simulink library "CCM_FVT"  (R2024a)
settings: Solver=VariableStepAuto  StartTime=0.0  StopTime=10.0  RelTol=1e-3
undefined symbols (not defined in the file or in its folder): ACCM_facCCMLq_X_A, ACCM_facCCMLq_Y_A, ACCM_facLPFiDAct_X_rpm, ACCM_IdKp_X_rpm, ACCM_tiCurErrOvr_X_A, CCM_bRstIpartTrig_C, CCM_bRstPIMor_C, CCM_bRstPITrig_C, CCM_bUseCCMVolFFTrig_C, CCM_bUseUvw_flg, CCM_facAngleComp, CCM_facCCMKiUdTar_T, CCM_facCCMKiUqTar_T, CCM_facCCMKpUdTar_T, CCM_facCCMKpUqTar_T, CCM_facCCMLd_T, CCM_facCCMLq_T, CCM_facLPFiDAct_T, CCM_facLPFiQAct_T, CCM_iCurrDQRstIntgl_C, CCM_iDCurrAct_A, CCM_iDErrDeadZoneLo_C, CCM_iDErrDeadZoneUp_C, CCM_iQErrDeadZoneLo_C, CCM_iQErrDeadZoneUp_C, CCM_nRotCCMKpKi_A, CCM_nRotRstIntgl_C, CCM_nRotSpdLPFiDQAct_A, CCM_uDVoltTarMax_C, CCM_uDVoltTarMin_C, CCM_uDVoltTarMor_C, CCM_uDVoltTarTrig_C, CCM_uQVoltTarMax_C, CCM_uQVoltTarMin_C, CCM_uQVoltTarMor_C, CCM_uQVoltTarTrig_C, CDC_iQCurrAct_A, CDC_tqMotCurrTarMTPV_A, ENUM_IVTROPMODE_DTCYCTRL, IvtrM_vVehPCM2SpdKpKiTar_A, KCCM_BattVolFilTi_fac, KCCM_bRstCurErrorOverThd_C, KCCM_CurLoopPrd_t, KCCM_FwdMask_c, KCCM_IdKi_null, KCCM_IdKp_null, KCCM_IdKt_null, KCCM_IqKi_null, KCCM_IqKp_null, KCCM_IqKt_null, KCCM_PosnRange_deg, KCCM_tiCurErrOvr_C, KCCM_UdqASCEna_C, KCCM_UdqASCTagValue_C, KCCM_UdqASCTimesValue_C, KCCM_VdSp_V, KCCM_VdSpSwEna_flg, KCCM_VolMod_perc, KCCM_VqSp_V, KDSM_CurErrorThd2_value ... (+33)
libraries: simulink x10, GRC_Lib x6, FVTMCU_lib x2
(part 1 of 2)
settings Model: Creator=FVT22063  LastModifiedBy=FVT22063

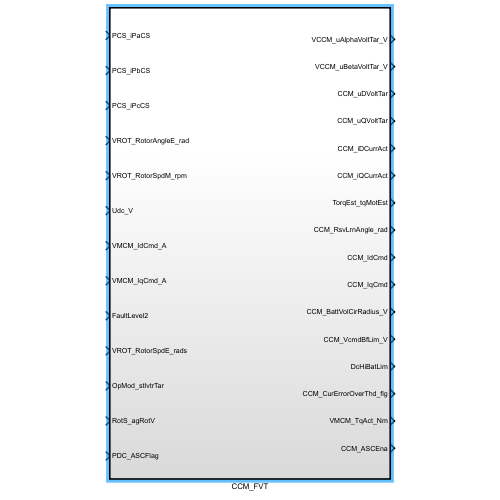
[thumbnail: Simulink's stored preview of the top-level diagram]
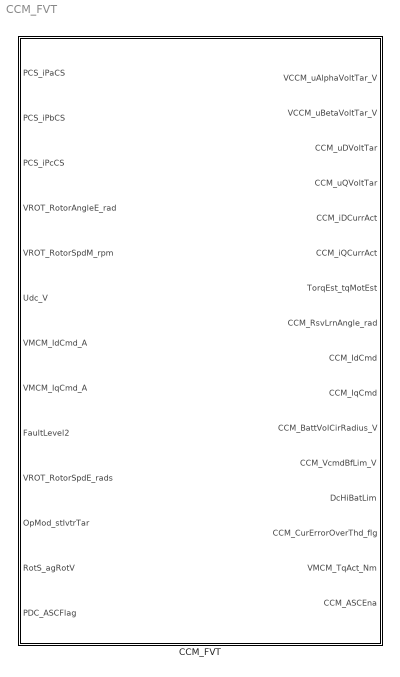
== system CCM_FVT ==
  CCM_FVT : Subsystem  TreatAsAtomicUnit=on
      settings: RTWSystemCode=Nonreusable function  RTWFcnNameOpts=Use subsystem name  RTWFileNameOpts=Use subsystem name

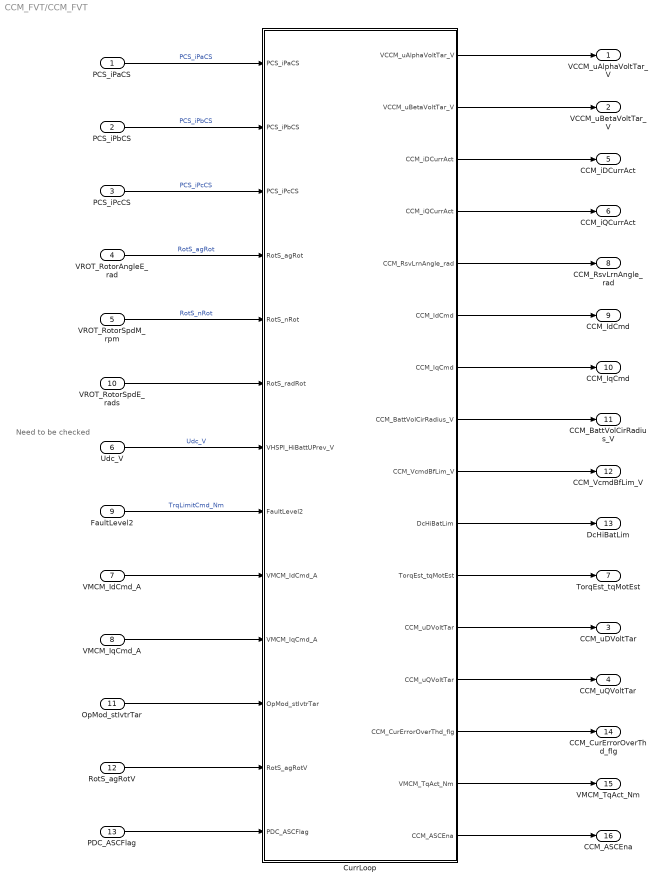
== system CCM_FVT/CCM_FVT ==
  note: Need to be checked
  PCS_iPaCS : Inport
  PCS_iPbCS : Inport  Port=2
  PCS_iPcCS : Inport  Port=3
  VROT_RotorAngleE_rad : Inport  Port=4
  VROT_RotorSpdM_rpm : Inport  Port=5
  Udc_V : Inport  Port=6
  VMCM_IdCmd_A : Inport  Port=7
  VMCM_IqCmd_A : Inport  Port=8
  FaultLevel2 : Inport  Port=9
  VROT_RotorSpdE_rads : Inport  Port=10
  OpMod_stIvtrTar : Inport  Port=11
  RotS_agRotV : Inport  Port=12
  PDC_ASCFlag : Inport  Port=13
  CurrLoop : Subsystem
  VCCM_uAlphaVoltTar_V : Outport  VectorParamsAs1DForOutWhenUnconnected=off
  VCCM_uBetaVoltTar_V : Outport  Port=2  VectorParamsAs1DForOutWhenUnconnected=off
  CCM_uDVoltTar : Outport  Port=3  VectorParamsAs1DForOutWhenUnconnected=off
  CCM_uQVoltTar : Outport  Port=4  VectorParamsAs1DForOutWhenUnconnected=off
  CCM_iDCurrAct : Outport  Port=5  VectorParamsAs1DForOutWhenUnconnected=off
  CCM_iQCurrAct : Outport  Port=6  VectorParamsAs1DForOutWhenUnconnected=off
  TorqEst_tqMotEst : Outport  Port=7  VectorParamsAs1DForOutWhenUnconnected=off
  CCM_RsvLrnAngle_rad : Outport  Port=8
  CCM_IdCmd : Outport  Port=9  VectorParamsAs1DForOutWhenUnconnected=off
  CCM_IqCmd : Outport  Port=10  VectorParamsAs1DForOutWhenUnconnected=off
  CCM_BattVolCirRadius_V : Outport  Port=11  VectorParamsAs1DForOutWhenUnconnected=off
  CCM_VcmdBfLim_V : Outport  Port=12  VectorParamsAs1DForOutWhenUnconnected=off
  DcHiBatLim : Outport  Port=13  VectorParamsAs1DForOutWhenUnconnected=off
  CCM_CurErrorOverThd_flg : Outport  Port=14  VectorParamsAs1DForOutWhenUnconnected=off
  VMCM_TqAct_Nm : Outport  Port=15  VectorParamsAs1DForOutWhenUnconnected=off
  CCM_ASCEna : Outport  Port=16  VectorParamsAs1DForOutWhenUnconnected=off
  wires:
  PCS_iPaCS/1 -> CurrLoop/1(PCS_iPaCS)  "PCS_iPaCS"
  PCS_iPbCS/1 -> CurrLoop/2(PCS_iPbCS)  "PCS_iPbCS"
  PCS_iPcCS/1 -> CurrLoop/3(PCS_iPcCS)  "PCS_iPcCS"
  VROT_RotorAngleE_rad/1 -> CurrLoop/4(RotS_agRot)  "RotS_agRot"
  VROT_RotorSpdM_rpm/1 -> CurrLoop/5(RotS_nRot)  "RotS_nRot"
  VROT_RotorSpdE_rads/1 -> CurrLoop/6(RotS_radRot)
  Udc_V/1 -> CurrLoop/7(VHSPI_HiBattUPrev_V)  "Udc_V"
  CurrLoop/1(VCCM_uAlphaVoltTar_V) -> VCCM_uAlphaVoltTar_V/1
  CurrLoop/2(VCCM_uBetaVoltTar_V) -> VCCM_uBetaVoltTar_V/1
  CurrLoop/3(CCM_iDCurrAct) -> CCM_iDCurrAct/1
  CurrLoop/4(CCM_iQCurrAct) -> CCM_iQCurrAct/1
  CurrLoop/5(CCM_RsvLrnAngle_rad) -> CCM_RsvLrnAngle_rad/1
  CurrLoop/6(CCM_IdCmd) -> CCM_IdCmd/1
  CurrLoop/7(CCM_IqCmd) -> CCM_IqCmd/1
  CurrLoop/11(TorqEst_tqMotEst) -> TorqEst_tqMotEst/1
  CurrLoop/12(CCM_uDVoltTar) -> CCM_uDVoltTar/1
  CurrLoop/13(CCM_uQVoltTar) -> CCM_uQVoltTar/1
  FaultLevel2/1 -> CurrLoop/8(FaultLevel2)  "TrqLimitCmd_Nm"
  VMCM_IdCmd_A/1 -> CurrLoop/9(VMCM_IdCmd_A)
  VMCM_IqCmd_A/1 -> CurrLoop/10(VMCM_IqCmd_A)
  OpMod_stIvtrTar/1 -> CurrLoop/11("OpMod_stIvtrTar ")
  RotS_agRotV/1 -> CurrLoop/12(RotS_agRotV)
  PDC_ASCFlag/1 -> CurrLoop/13("PDC_ASCFlag ")
  CurrLoop/8(CCM_BattVolCirRadius_V) -> CCM_BattVolCirRadius_V/1
  CurrLoop/9(CCM_VcmdBfLim_V) -> CCM_VcmdBfLim_V/1
  CurrLoop/10(DcHiBatLim) -> DcHiBatLim/1
  CurrLoop/14(CCM_CurErrorOverThd_flg) -> CCM_CurErrorOverThd_flg/1
  CurrLoop/15(VMCM_TqAct_Nm) -> VMCM_TqAct_Nm/1
  CurrLoop/16("CCM_ASCEna ") -> CCM_ASCEna/1

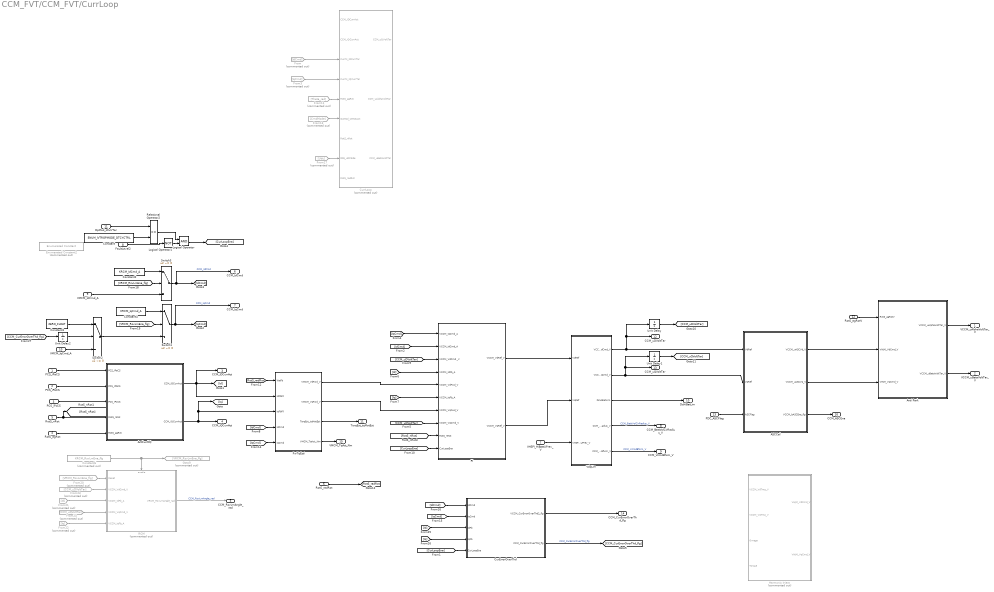
== system CCM_FVT/CCM_FVT/CurrLoop ==
  PCS_iPaCS : Inport  OutDataTypeStr=single
  PCS_iPbCS : Inport  Port=2  OutDataTypeStr=single
  PCS_iPcCS : Inport  Port=3  OutDataTypeStr=single
  RotS_agRot : Inport  Port=4  OutDataTypeStr=single
  RotS_nRot : Inport  Port=5  OutDataTypeStr=single
  RotS_radRot : Inport  Port=6
  VHSPI_HiBattUPrev_V : Inport  Port=7  OutDataTypeStr=single
  FaultLevel2 : Inport  Port=8
  VMCM_IdCmd_A : Inport  Port=9  OutDataTypeStr=single
  VMCM_IqCmd_A : Inport  Port=10  OutDataTypeStr=single
  "OpMod_stIvtrTar " : Inport  Port=11
  RotS_agRotV : Inport  Port=12  OutDataTypeStr=single
  "PDC_ASCFlag " : Inport  Port=13
  ASCCal : Subsystem
  ActCurrDQ : Subsystem
  Anti Park : Subsystem
  Constant : Constant  Value=ENUM_IVTROPMODE_DTCYCTRL
  Constant2 : Constant  Value=KRCM_IdCmd_A
  Constant3 : Constant  Value=ZERO_FLOAT
  Constant4 : Constant  Value=KRCM_IqCmd_A
  Constant6 : Constant  Commented=on  Value=KRCM_RsvLrnEna_flg  SampleTime=-1
  CurErrorOverThd : Subsystem
  CurrLoop : Subsystem  Commented=on
  Enumerated Constant2 : simulink/Sources/Enumerated Constant  Commented=on  OutDataTypeStr=Enum: StIvtrMod  Value=StIvtrMod.StIvtrModDtcyCtrl  SampleTime=inf
  From : From  Commented=on  GotoTag=IdCmd
  From11 : From  Commented=on  GotoTag=Theta_rad
  From13 : From  Commented=on  GotoTag=CmdMode
  From17 : From  Commented=on  GotoTag=Udc
  From20 : From  Commented=on  GotoTag=VRCM_RsvLrnEna_flg
  From21 : From  Commented=on  GotoTag=Id
  From22 : From  Commented=on  GotoTag=Iq
  From23 : From  Commented=on  GotoTag=CCM_uDVoltTar
  From24 : From  Commented=on  GotoTag=CCM_uQVoltTar
  From3 : From  Commented=on  GotoTag=IqCmd
  FwTqEsti : Subsystem
  Goto9 : Goto  Commented=on  GotoTag=VRCM_RsvLrnEna_flg
  Harmonic Inject : Subsystem  Commented=on
  Logical Operator : Logic  AllPortsSameDT=off  OutDataTypeStr=boolean
  Logical Operator1 : Logic  Operator=NOT  AllPortsSameDT=off  OutDataTypeStr=boolean
  PI : Subsystem
  RCM : Subsystem  Commented=on
  Relational Operator2 : RelationalOperator  Operator===  OutDataTypeStr=boolean  RndMeth=Simplest  InputSameDT=off
  Switch1 : Switch  Criteria=u2 ~= 0  SaturateOnIntegerOverflow=off  InputSameDT=off
  Switch2 : Switch  Criteria=u2 ~= 0  SaturateOnIntegerOverflow=off  InputSameDT=off
  Switch3 : Switch  Criteria=u2 ~= 0  SaturateOnIntegerOverflow=off  InputSameDT=off
  Unit Delay : UnitDelay  SampleTime=-1  HasFrameUpgradeWarning=on
  Unit Delay1 : UnitDelay  SampleTime=-1  HasFrameUpgradeWarning=on
  Unit Delay2 : UnitDelay  SampleTime=-1  HasFrameUpgradeWarning=on
  VdqLim : Subsystem
  VCCM_uAlphaVoltTar_V : Outport  OutDataTypeStr=single  VectorParamsAs1DForOutWhenUnconnected=off
  VCCM_uBetaVoltTar_V : Outport  Port=2  OutDataTypeStr=single  VectorParamsAs1DForOutWhenUnconnected=off
  CCM_iDCurrAct : Outport  Port=3  OutDataTypeStr=single  VectorParamsAs1DForOutWhenUnconnected=off
  CCM_iQCurrAct : Outport  Port=4  OutDataTypeStr=single  VectorParamsAs1DForOutWhenUnconnected=off
  CCM_RsvLrnAngle_rad : Outport  Port=5  OutDataTypeStr=single
  CCM_IdCmd : Outport  Port=6  OutDataTypeStr=single  VectorParamsAs1DForOutWhenUnconnected=off
  CCM_IqCmd : Outport  Port=7  OutDataTypeStr=single  VectorParamsAs1DForOutWhenUnconnected=off
  CCM_BattVolCirRadius_V : Outport  Port=8  OutDataTypeStr=single
  CCM_VcmdBfLim_V : Outport  Port=9  OutDataTypeStr=single
  DcHiBatLim : Outport  Port=10
  TorqEst_tqMotEst : Outport  Port=11  OutDataTypeStr=single  VectorParamsAs1DForOutWhenUnconnected=off
  CCM_uDVoltTar : Outport  Port=12  VectorParamsAs1DForOutWhenUnconnected=off
  CCM_uQVoltTar : Outport  Port=13  VectorParamsAs1DForOutWhenUnconnected=off
  CCM_CurErrorOverThd_flg : Outport  Port=14  VectorParamsAs1DForOutWhenUnconnected=off
  VMCM_TqAct_Nm : Outport  Port=15
  "CCM_ASCEna " : Outport  Port=16  VectorParamsAs1DForOutWhenUnconnected=off
  wires:
  PCS_iPaCS/1 -> ActCurrDQ/1(PCS_iPaCS)
  PCS_iPbCS/1 -> ActCurrDQ/2(PCS_iPbCS)
  PCS_iPcCS/1 -> ActCurrDQ/3(PCS_iPcCS)
  RotS_agRot/1 -> ActCurrDQ/5(RotS_agRot)
  RotS_nRot/1 -> [RotS_nRot], ActCurrDQ/4(RotS_nRot)
  From13/1 -> CurrLoop/6(OpMod_stMotAct)
  From/1 -> CurrLoop/3(CurrM_iDCurrTar)
  From3/1 -> CurrLoop/4(CurrM_iQCurrTar)
  [RotS_nRot] -> PI/9(RotS_nRot)
  From11/1 -> CurrLoop/5(RotS_agRot)
  Switch1/1 -> CCM_IqCmd/1, [IqCmd]  "CCM_IqCmd"
  From17/1 -> CurrLoop/8(DSS_uDCSide)
  Switch3/1 -> CCM_IdCmd/1, [IdCmd]  "CCM_IdCmd"
  Constant2/1 -> Switch3/1
  [VRCM_RsvLrnEna_flg] -> Switch3/2
  [VRCM_RsvLrnEna_flg] -> Switch1/2
  Constant4/1 -> Switch1/1
  Constant6/1 -> Goto9/1, RCM/Enable
  From20/1 -> RCM/1("Reset ")
  From22/1 -> RCM/5("VCCM_IqFb_A ")
  From21/1 -> RCM/3("VCCM_IdFb_A ")
  From23/1 -> RCM/2("VCCM_VdCmd_V ")
  From24/1 -> RCM/4("VCCM_VqCmd_V ")
  Unit Delay/1 -> [CCM_uDVoltTar]
  Unit Delay1/1 -> [CCM_uQVoltTar]
  RCM/1("VRCM_RsvLrnAngle_rad ") -> CCM_RsvLrnAngle_rad/1  "CCM_RsvLrnAngle_rad"
  PI/1(VCCM_VdRef_V) -> VdqLim/1(VdRef)
  VdqLim/4(CCM_BattVolCirRadius_V) -> CCM_BattVolCirRadius_V/1  "CCM_BattVolCirRadius_V"
  PI/2(VCCM_VqRef_V) -> VdqLim/2(VqRef)
  VdqLim/5(CCM_VcmdBfLim_V) -> CCM_VcmdBfLim_V/1  "CCM_VcmdBfLim_V"
  VdqLim/2(VCCM_VqCmd_V) -> ASCCal/2(VqRef), Unit Delay1/1, CCM_uQVoltTar/1
  VHSPI_HiBattUPrev_V/1 -> VdqLim/3(VHSPI_HiBattUPrev_V)
  ActCurrDQ/1(CCM_iDCurrAct) -> FwTqEsti/2(IdFbFil), [Id], CCM_iDCurrAct/1
  ActCurrDQ/2(CCM_iQCurrAct) -> [Iq], FwTqEsti/3(IqFbFil), CCM_iQCurrAct/1
  [IdCmd] -> PI/2(VCCM_IdCmd_A)
  [IqCmd] -> PI/1(VCCM_IqCmd_A)
  VMCM_IdCmd_A/1 -> Switch3/3
  RotS_radRot/1 -> [RotS_radRot]
  "OpMod_stIvtrTar "/1 -> Relational Operator2/1
  VdqLim/3(DcHiBatLim) -> DcHiBatLim/1
  RotS_agRotV/1 -> Anti Park/1(RotS_agRotV)
  Anti Park/1(VCCM_uAlphaVoltTar_V) -> VCCM_uAlphaVoltTar_V/1
  Anti Park/2(VCCM_uBetaVoltTar_V) -> VCCM_uBetaVoltTar_V/1
  VdqLim/1(VCCM_VdCmd_V) -> Unit Delay/1, CCM_uDVoltTar/1, ASCCal/1(VdRef)
  [Id] -> PI/4(VCCM_IdFb_A)
  [Iq] -> PI/6(VCCM_IqFb_A)
  [CCM_uDVoltTar] -> PI/3(VCCM_VdCmd _V)
  [CCM_uQVoltTar] -> PI/8(VCCM_VqCmd_V)
  FaultLevel2/1 -> Logical Operator1/1
  [RotS_radRot] -> FwTqEsti/1(WeFb)
  FwTqEsti/1(VMCM_VdFwd_V) -> PI/5(VCCM_VdFwd_V)
  FwTqEsti/2(VMCM_VqFwd_V) -> PI/7(VCCM_VqFwd_V)
  [IdCmd] -> FwTqEsti/4(IdCmd)
  [IqCmd] -> FwTqEsti/5(IqCmd)
  FwTqEsti/3(TorqEst_tqMotEst) -> TorqEst_tqMotEst/1
  Relational Operator2/1 -> Logical Operator/1
  Logical Operator1/1 -> Logical Operator/2
  Logical Operator/1 -> [CurLoopEna]
  [CurLoopEna] -> CurErrorOverThd/5(CurLoopEna)
  [CurLoopEna] -> PI/10(CurLoopEna)
  [IdCmd] -> CurErrorOverThd/1(IdCmd)
  [IqCmd] -> CurErrorOverThd/2(IqCmd)
  [Iq] -> CurErrorOverThd/4(IqFb)
  [Id] -> CurErrorOverThd/3(IdFb)
  FwTqEsti/4(VMCM_TqAct_Nm) -> VMCM_TqAct_Nm/1
  ASCCal/1(VCCM_uASCVd_V) -> Anti Park/2(VHJM_VdCmd_V)
  ASCCal/2(VCCM_uASCVq_V) -> Anti Park/3(VHJM_VqCmd_V)
  ASCCal/3("VCCM_bASCEna_flg ") -> "CCM_ASCEna "/1
  "PDC_ASCFlag "/1 -> ASCCal/3("ASCFlag ")
  Constant/1 -> Relational Operator2/2
  Unit Delay2/1 -> Switch2/2
  [CCM_CurErrorOverThd_flg] -> Unit Delay2/1
  Constant3/1 -> Switch2/1
  VMCM_IqCmd_A/1 -> Switch2/3
  Switch2/1 -> Switch1/3
  CurErrorOverThd/1(VCCM_CurErrorOverThd2_flg) -> CCM_CurErrorOverThd_flg/1
  CurErrorOverThd/2(CCM_CurErrorOverThd_flg) -> [CCM_CurErrorOverThd_flg]  "CCM_CurErrorOverThd_flg"

== system CCM_FVT/CCM_FVT/CurrLoop/ASCCal ==
  VdRef : Inport
  VqRef : Inport  Port=2
  "ASCFlag " : Inport  Port=3
  Constant2 : Constant  Value=KCCM_UdqASCEna_C
  If : If  IfExpression=u1 ~= 0
  If Action Subsystem : Subsystem  TreatAsAtomicUnit=on
  Merge : Merge
  Merge1 : Merge
  Merge2 : Merge
  Signal Conversion : SignalConversion  OverrideOpt=off
  Subsystem1 : Subsystem
  VCCM_uASCVd_V : Outport
  VCCM_uASCVq_V : Outport  Port=2
  "VCCM_bASCEna_flg " : Outport  Port=3
  wires:
  VqRef/1 -> If Action Subsystem/2(VqRef), Subsystem1/2(VqRef)
  Constant2/1 -> If/1
  VdRef/1 -> If Action Subsystem/1(VdRef), Subsystem1/1(VdRef)
  Merge/1 -> VCCM_uASCVd_V/1  "VCCM_uASCVd_V"
  Merge2/1 -> Signal Conversion/1  "CCM_bASCEna"
  Merge1/1 -> VCCM_uASCVq_V/1  "VCCM_uASCVq_V"
  "ASCFlag "/1 -> If Action Subsystem/3(ASCFlag), Subsystem1/3("ASCFlag ")
  If/1 -> Subsystem1/Action
  If/2 -> If Action Subsystem/Action
  If Action Subsystem/3(enASC_flg) -> Merge2/2
  If Action Subsystem/2(Vq) -> Merge1/2
  If Action Subsystem/1(Vd) -> Merge/2
  Subsystem1/3(enASC_flg) -> Merge2/1
  Subsystem1/2(Vq) -> Merge1/1
  Subsystem1/1(Vd) -> Merge/1
  Signal Conversion/1 -> "VCCM_bASCEna_flg "/1  "VCCM_bASCEna_flg"

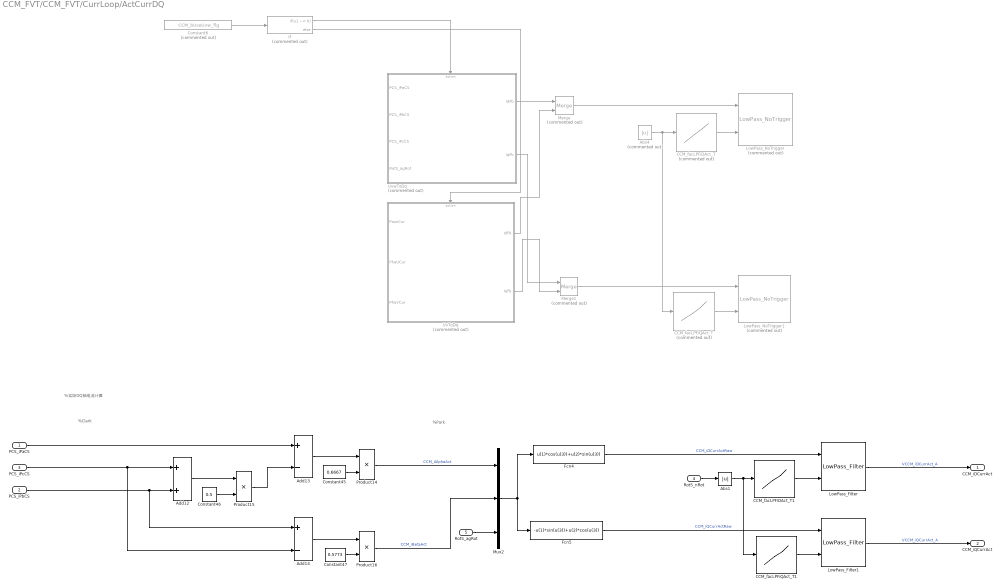
== system CCM_FVT/CCM_FVT/CurrLoop/ActCurrDQ ==
  note: %Clark
  note: %Park
  note: %实际DQ轴电流计算
  PCS_iPaCS : Inport  OutDataTypeStr=single
  PCS_iPbCS : Inport  Port=2  OutDataTypeStr=single
  PCS_iPcCS : Inport  Port=3  OutDataTypeStr=single
  RotS_nRot : Inport  Port=4  OutDataTypeStr=single
  RotS_agRot : Inport  Port=5  OutDataTypeStr=single
  Abs1 : Abs  SaturateOnIntegerOverflow=off
  Abs4 : Abs  Commented=on  SaturateOnIntegerOverflow=off
  Add12 : Sum
  Add13 : Sum  Inputs=+-
  Add14 : Sum  Inputs=+-
  CCM_facLPFiDAct_T : Lookup_n-D  Commented=on  NumberOfTableDimensions=1  BreakpointsForDimension1=CCM_nRotSpdLPFiDQAct_A  BreakpointsForDimension2=IvtrM_vVehPCM2SpdKpKiTar_A  Table=CCM_facLPFiDAct_T  TableDataTypeStr=Inherit: Inherit from 'Table data'  ExtrapMethod=Clip  UseLastTableValue=on  InternalRulePriority=Speed  OutDataTypeStr=Inherit: Inherit from 'Table data'  RndMeth=Simplest  InputSameDT=off
  CCM_facLPFiDAct_T1 : Lookup_n-D  NumberOfTableDimensions=1  BreakpointsForDimension1=ACCM_facLPFiDAct_X_rpm  BreakpointsForDimension2=IvtrM_vVehPCM2SpdKpKiTar_A  Table=MCCM_facLPFiDAct_Y_T  TableDataTypeStr=Inherit: Inherit from 'Table data'  ExtrapMethod=Clip  UseLastTableValue=on  InternalRulePriority=Speed  OutDataTypeStr=Inherit: Inherit from 'Table data'  RndMeth=Simplest  InputSameDT=off
  CCM_facLPFiQAct_T : Lookup_n-D  Commented=on  NumberOfTableDimensions=1  BreakpointsForDimension1=CCM_nRotSpdLPFiDQAct_A  BreakpointsForDimension2=IvtrM_vVehPCM2SpdKpKiTar_A  Table=CCM_facLPFiQAct_T  TableDataTypeStr=Inherit: Inherit from 'Table data'  ExtrapMethod=Clip  UseLastTableValue=on  InternalRulePriority=Speed  OutDataTypeStr=Inherit: Inherit from 'Table data'  RndMeth=Simplest  InputSameDT=off
  CCM_facLPFiQAct_T1 : Lookup_n-D  NumberOfTableDimensions=1  BreakpointsForDimension1=ACCM_facLPFiDAct_X_rpm  BreakpointsForDimension2=IvtrM_vVehPCM2SpdKpKiTar_A  Table=MCCM_facLPFiQAct_Y_T  TableDataTypeStr=Inherit: Inherit from 'Table data'  ExtrapMethod=Clip  UseLastTableValue=on  InternalRulePriority=Speed  OutDataTypeStr=Inherit: Inherit from 'Table data'  RndMeth=Simplest  InputSameDT=off
  Constant45 : Constant  Value=0.6667  OutDataTypeStr=single
  Constant46 : Constant  Value=0.5  OutDataTypeStr=single
  Constant47 : Constant  Value=0.5773  OutDataTypeStr=single
  Constant6 : Constant  Commented=on  Value=CCM_bUseUvw_flg  SampleTime=-1
  Fcn4 : Fcn  Expr=u(1)*cos(u(3))+u(2)*sin(u(3))
  Fcn5 : Fcn  Expr=-u(1)*sin(u(3))+u(2)*cos(u(3))
  If : If  Commented=on  IfExpression=u1 ~= 0
  LowPass_Filter : FVTMCU_lib/LowPass_Filter  SystemSampleTime=-1  VariantActivationTime=update diagram  AllowFlexibleInterface=on  Latency=0  AutoFrameSizeCalculation=off
  LowPass_Filter1 : FVTMCU_lib/LowPass_Filter  SystemSampleTime=-1  VariantActivationTime=update diagram  AllowFlexibleInterface=on  Latency=0  AutoFrameSizeCalculation=off
  LowPass_NoTrigger : GRC_Lib/Filter/LowPass_NoTrigger  Commented=on  IpDT=single
  LowPass_NoTrigger1 : GRC_Lib/Filter/LowPass_NoTrigger  Commented=on  IpDT=single
  Merge : Merge  Commented=on
  Merge1 : Merge  Commented=on
  Mux2 : Mux  Inputs=3
  Product14 : Product
  Product15 : Product
  Product16 : Product
  UvToDq : Subsystem  Commented=on
  UvwToDq : Subsystem  Commented=on
  CCM_iDCurrAct : Outport  OutDataTypeStr=single  VectorParamsAs1DForOutWhenUnconnected=off
  CCM_iQCurrAct : Outport  Port=2  OutDataTypeStr=single  VectorParamsAs1DForOutWhenUnconnected=off
  wires:
  Abs4/1 -> CCM_facLPFiQAct_T/1, CCM_facLPFiDAct_T/1
  CCM_facLPFiQAct_T/1 -> LowPass_NoTrigger1/2
  CCM_facLPFiDAct_T/1 -> LowPass_NoTrigger/2
  Constant6/1 -> If/1
  If/1 -> UvwToDq/Action
  If/2 -> UvToDq/Action
  UvwToDq/1(IdFb) -> Merge/1
  UvToDq/1(IdFb) -> Merge/2
  UvwToDq/2(IqFb) -> Merge1/1
  UvToDq/2(IqFb) -> Merge1/2
  Merge/1 -> LowPass_NoTrigger/1
  Merge1/1 -> LowPass_NoTrigger1/1
  Constant46/1 -> Product15/2
  CCM_facLPFiDAct_T1/1 -> LowPass_Filter/2
  Mux2/1 -> Fcn5/1, Fcn4/1
  LowPass_Filter/1 -> CCM_iDCurrAct/1  "VCCM_iDCurrAct_A"
  CCM_facLPFiQAct_T1/1 -> LowPass_Filter1/2
  Add12/1 -> Product15/1
  Product15/1 -> Add13/2
  Fcn5/1 -> LowPass_Filter1/1  "CCM_iQCurrActRaw"
  Constant47/1 -> Product16/2
  Product16/1 -> Mux2/2  "CCM_iBetaAct"
  Add14/1 -> Product16/1
  Constant45/1 -> Product14/2
  PCS_iPbCS/1 -> Add14/1, Add12/2
  Fcn4/1 -> LowPass_Filter/1  "CCM_iDCurrActRaw"
  RotS_agRot/1 -> Mux2/3
  PCS_iPcCS/1 -> Add14/2, Add12/1
  PCS_iPaCS/1 -> Add13/1
  Add13/1 -> Product14/1
  Product14/1 -> Mux2/1  "CCM_iAlphaAct"
  Abs1/1 -> CCM_facLPFiQAct_T1/1, CCM_facLPFiDAct_T1/1
  RotS_nRot/1 -> Abs1/1
  LowPass_Filter1/1 -> CCM_iQCurrAct/1  "VCCM_iQCurrAct_A"

== system CCM_FVT/CCM_FVT/CurrLoop/Anti Park ==
  note: %转子角度
  note: %Anti-Park
  RotS_agRotV : Inport  OutDataTypeStr=single
  VHJM_VdCmd_V : Inport  Port=2
  VHJM_VqCmd_V : Inport  Port=3
  Fcn : Fcn  Expr=cos(u[1])*u[2]-sin(u[1])*u[3]
  Fcn1 : Fcn  Expr=sin(u[1])*u[2]+cos(u[1])*u[3]
  Mux : Mux  Inputs=3
  VCCM_uAlphaVoltTar_V : Outport  OutDataTypeStr=single  VectorParamsAs1DForOutWhenUnconnected=off
  VCCM_uBetaVoltTar_V : Outport  Port=2  OutDataTypeStr=single  VectorParamsAs1DForOutWhenUnconnected=off
  wires:
  VHJM_VdCmd_V/1 -> Mux/2
  Fcn1/1 -> VCCM_uBetaVoltTar_V/1  "VCCM_uBetaVoltTar_V"
  Fcn/1 -> VCCM_uAlphaVoltTar_V/1  "VCCM_uAlphaVoltTar_V"
  VHJM_VqCmd_V/1 -> Mux/3
  Mux/1 -> Fcn/1, Fcn1/1
  RotS_agRotV/1 -> Mux/1

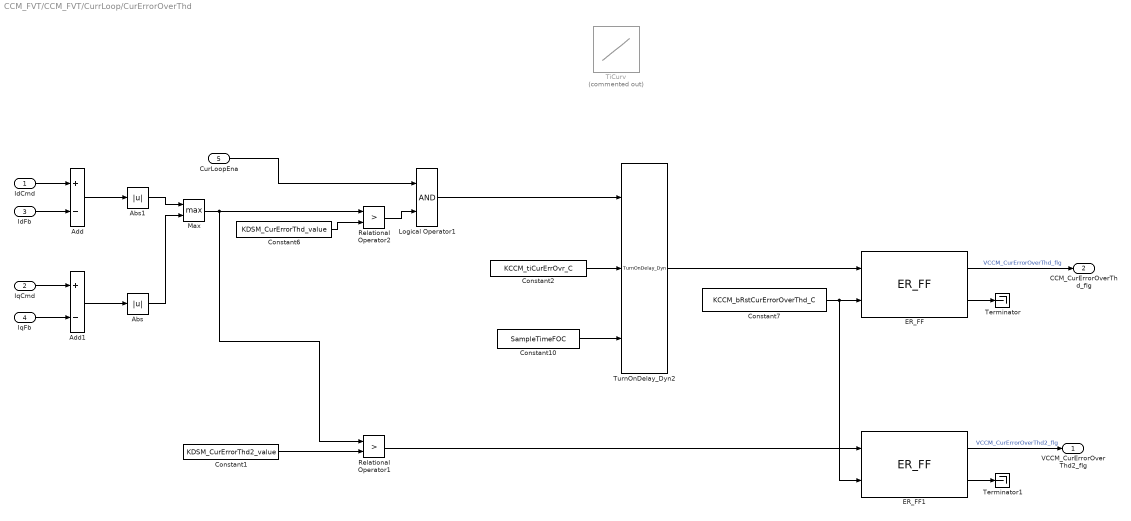
== system CCM_FVT/CCM_FVT/CurrLoop/CurErrorOverThd ==
  IdCmd : Inport
  IqCmd : Inport  Port=2
  IdFb : Inport  Port=3
  IqFb : Inport  Port=4
  CurLoopEna : Inport  Port=5
  Abs : Abs  SaturateOnIntegerOverflow=off
  Abs1 : Abs  SaturateOnIntegerOverflow=off
  Add : Sum  Inputs=+-
  Add1 : Sum  Inputs=+-
  Constant1 : Constant  Value=KDSM_CurErrorThd2_value
  Constant10 : Constant  Value=SampleTimeFOC
  Constant2 : Constant  Value=KCCM_tiCurErrOvr_C
  Constant6 : Constant  Value=KDSM_CurErrorThd_value
  Constant7 : Constant  Value=KCCM_bRstCurErrorOverThd_C
  ER_FF : GRC_Lib/Memory/ER_FF  FalseVal=0  TrueVal=1
  ER_FF1 : GRC_Lib/Memory/ER_FF  FalseVal=0  TrueVal=1
  Logical Operator1 : Logic  AllPortsSameDT=off  OutDataTypeStr=boolean
  Max : MinMax  Function=max  Inputs=2
  Relational Operator1 : RelationalOperator  Operator=>  OutDataTypeStr=boolean  RndMeth=Simplest  InputSameDT=off
  Relational Operator2 : RelationalOperator  Operator=>  OutDataTypeStr=boolean  RndMeth=Simplest  InputSameDT=off
  Terminator : Terminator
  Terminator1 : Terminator
  "TiCurv " : Lookup_n-D  Commented=on  NumberOfTableDimensions=1  BreakpointsForDimension1=ACCM_tiCurErrOvr_X_A  Table=MCCM_tiCurErrOvr_Y_T  ExtrapMethod=Clip  UseLastTableValue=on  InternalRulePriority=Speed  RndMeth=Simplest
  TurnOnDelay_Dyn2 : GRC_Lib/Delay/TurnOnDelay_Dyn  IpDT=single
  VCCM_CurErrorOverThd2_flg : Outport  VectorParamsAs1DForOutWhenUnconnected=off
  CCM_CurErrorOverThd_flg : Outport  Port=2  VectorParamsAs1DForOutWhenUnconnected=off
  wires:
  IdCmd/1 -> Add/1
  Add1/1 -> Abs/1
  Constant6/1 -> Relational Operator2/2
  Abs/1 -> Max/2
  Add/1 -> Abs1/1
  Abs1/1 -> Max/1
  ER_FF/1 -> CCM_CurErrorOverThd_flg/1  "VCCM_CurErrorOverThd_flg"
  Relational Operator2/1 -> Logical Operator1/2
  CurLoopEna/1 -> Logical Operator1/1
  IdFb/1 -> Add/2
  IqCmd/1 -> Add1/1
  IqFb/1 -> Add1/2
  Logical Operator1/1 -> TurnOnDelay_Dyn2/1
  Constant7/1 -> ER_FF1/2, ER_FF/2
  Constant10/1 -> TurnOnDelay_Dyn2/3
  TurnOnDelay_Dyn2/1 -> ER_FF/1
  ER_FF/2 -> Terminator/1
  Constant1/1 -> Relational Operator1/2
  Max/1 -> Relational Operator2/1, Relational Operator1/1
  Relational Operator1/1 -> ER_FF1/1
  Constant2/1 -> TurnOnDelay_Dyn2/2
  ER_FF1/2 -> Terminator1/1
  ER_FF1/1 -> VCCM_CurErrorOverThd2_flg/1  "VCCM_CurErrorOverThd2_flg"

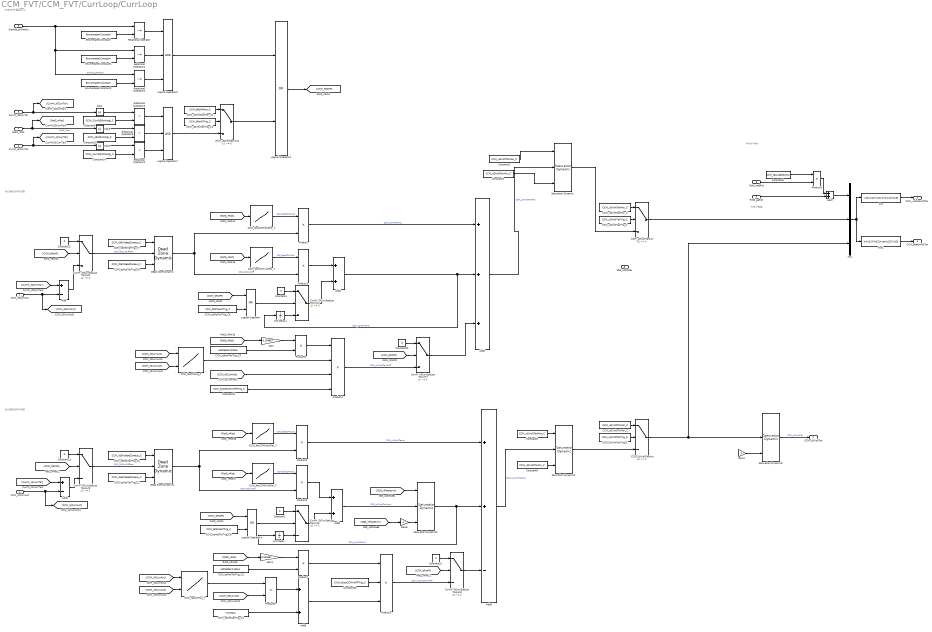
== system CCM_FVT/CCM_FVT/CurrLoop/CurrLoop ==
  note: %转子角度
  note: %电流环PI重置条件
  note: %Q轴电流环PI控制
  note: %D轴电流环PI控制
  note: %Anti-Park
  CCM_iDCurrAct : Inport  OutDataTypeStr=single
  CCM_iQCurrAct : Inport  Port=2  OutDataTypeStr=single
  CurrM_iDCurrTar : Inport  Port=3  OutDataTypeStr=single
  CurrM_iQCurrTar : Inport  Port=4  OutDataTypeStr=single
  RotS_agRot : Inport  Port=5  OutDataTypeStr=single
  OpMod_stMotAct : Inport  Port=6  OutDataTypeStr=Enum: StMotMod
  RotS_nRot : Inport  Port=7  OutDataTypeStr=single
  DSS_uDCSide : Inport  Port=8  OutDataTypeStr=single
  RotS_radRot : Inport  Port=9  OutDataTypeStr=single
  Abs1 : Abs  SaturateOnIntegerOverflow=off
  Abs2 : Abs  SaturateOnIntegerOverflow=off
  Abs3 : Abs  SaturateOnIntegerOverflow=off
  Add : Sum  Inputs=+-
  Add{1,4,6..7} (4 alike) : Sum
  Add2 : Sum  Inputs=+++
  Add3 : Sum  Inputs=+-
  Add5 : Sum  Inputs=++-
  CCM_facCCMKiUdTar_T : Lookup_n-D  NumberOfTableDimensions=1  BreakpointsForDimension1=CCM_nRotCCMKpKi_A  BreakpointsForDimension2=CDC_tqMotCurrTarMTPV_A  Table=CCM_facCCMKiUdTar_T  ExtrapMethod=Clip  UseLastTableValue=on  InternalRulePriority=Speed  RndMeth=Simplest
  CCM_facCCMKiUqTar_T : Lookup_n-D  NumberOfTableDimensions=1  BreakpointsForDimension1=CCM_nRotCCMKpKi_A  BreakpointsForDimension2=CDC_tqMotCurrTarMTPV_A  Table=CCM_facCCMKiUqTar_T  ExtrapMethod=Clip  UseLastTableValue=on  InternalRulePriority=Speed  RndMeth=Simplest
  CCM_facCCMKpUdTar_T : Lookup_n-D  NumberOfTableDimensions=1  BreakpointsForDimension1=CCM_nRotCCMKpKi_A  BreakpointsForDimension2=CDC_tqMotCurrTarMTPV_A  Table=CCM_facCCMKpUdTar_T  ExtrapMethod=Clip  UseLastTableValue=on  InternalRulePriority=Speed  RndMeth=Simplest
  CCM_facCCMKpUqTar_T : Lookup_n-D  NumberOfTableDimensions=1  BreakpointsForDimension1=CCM_nRotCCMKpKi_A  BreakpointsForDimension2=CDC_tqMotCurrTarMTPV_A  Table=CCM_facCCMKpUqTar_T  ExtrapMethod=Clip  UseLastTableValue=on  InternalRulePriority=Speed  RndMeth=Simplest
  CCM_facCCMLd_T : Lookup_n-D  BreakpointsForDimension1=CCM_iDCurrAct_A  BreakpointsForDimension2=CDC_iQCurrAct_A  Table=CCM_facCCMLd_T  ExtrapMethod=Clip  UseLastTableValue=on  InternalRulePriority=Speed  RndMeth=Simplest
      settings: InputPortMap=u0,u1
  CCM_facCCMLq_T : Lookup_n-D  BreakpointsForDimension1=CCM_iDCurrAct_A  BreakpointsForDimension2=CDC_iQCurrAct_A  Table=CCM_facCCMLq_T  ExtrapMethod=Clip  UseLastTableValue=on  InternalRulePriority=Speed  RndMeth=Simplest
      settings: InputPortMap=u0,u1
  CCM_tqMotTarTrig_C1 : Constant  Value=CCM_iQErrDeadZoneUp_C
  CCM_tqMotTarTrig_C2 : Constant  Value=CCM_iQErrDeadZoneLo_C
  CCM_tqMotTarTrig_C3 : Constant  Value=noPolePairs100us
  CCM_tqMotTarTrig_C4 : Constant  Value=Ym100us
  CCM_tqMotTarTrig_C5 : Constant  Value=noPolePairs100us
  CCM_tqMotTarTrig_C6 : Constant  Value=CCM_bRstIpartTrig_C
  CCM_tqMotTarTrig_C7 : Constant  Value=CCM_iDErrDeadZoneUp_C
  CCM_tqMotTarTrig_C8 : Constant  Value=CCM_iDErrDeadZoneLo_C
  CCM_tqMotTarTrig_C9 : Constant  Value=CCM_bRstIpartTrig_C
  CCM_uDVoltTarMor_C : Constant  Value=CCM_uDVoltTarMor_C
  CCM_uDVoltTarMor_C1 : Constant  Value=CCM_bRstPIMor_C
  CCM_uDVoltTarTrig_C : Constant  Value=CCM_uDVoltTarTrig_C
  CCM_uDVoltTarTrig_C1 : Constant  Value=CCM_bRstPITrig_C
  CCM_uDVoltTarswt : Switch  Criteria=u2 ~= 0  SaturateOnIntegerOverflow=off  InputSameDT=off
  CCM_uDVoltTarswt1 : Switch  Criteria=u2 ~= 0  SaturateOnIntegerOverflow=off  InputSameDT=off
  CCM_uQVoltTarMor_C : Constant  Value=CCM_uQVoltTarMor_C
  CCM_uQVoltTarTrig_C : Constant  Value=CCM_uQVoltTarTrig_C
  CCM_uQVoltTarswt : Switch  Criteria=u2 ~= 0  SaturateOnIntegerOverflow=off  InputSameDT=off
  Constant{1,4,12..13,21..22} (6 alike) : Constant  Value=0  OutDataTypeStr=single
  Constant14 : Constant  Value=CCM_iCurrDQRstIntgl_C
  Constant15 : Constant  Value=CCM_nRotRstIntgl_C
  Constant17 : Constant  Value=CCM_bUseCCMVolFFTrig_C
  Constant19 : Constant  Value=CCM_bUseCCMVolFFTrig_C
  Constant2 : Constant  Value=CCM_uDVoltTarMax_C
  Constant3 : Constant  Value=CCM_uDVoltTarMin_C
  Constant5 : Constant  Value=CCM_iCurrDQRstIntgl_C
  Constant6 : Constant  Value=CCM_facAngleComp  OutDataTypeStr=single
  Constant8 : Constant  Value=CCM_uQVoltTarMax_C
  Constant9 : Constant  Value=CCM_uQVoltTarMin_C
  CurrM_iDCurrSpdLopTarswt{1..4,6..7} (6 alike) : Switch  Criteria=u2 ~= 0  SaturateOnIntegerOverflow=off  InputSameDT=off
  Dead Zone Dynamic : simulink/Discontinuities/Dead Zone Dynamic
  Dead Zone Dynamic1 : simulink/Discontinuities/Dead Zone Dynamic
  Enumerated Constant : simulink/Sources/Enumerated Constant  OutDataTypeStr=Enum: StMotMod  Value=StMotMod.StMotModTqCtrl  SampleTime=inf
  Enumerated Constant1 : simulink/Sources/Enumerated Constant  OutDataTypeStr=Enum: StMotMod  Value=StMotMod.StMotModSpdCtrl  SampleTime=inf
  Enumerated Constant2 : simulink/Sources/Enumerated Constant  OutDataTypeStr=Enum: StMotMod  Value=StMotMod.StMotModDischarge  SampleTime=inf
  Fcn : Fcn  Expr=cos(u[1])*u[2]-sin(u[1])*u[3]
  Fcn1 : Fcn  Expr=sin(u[1])*u[2]+cos(u[1])*u[3]
  Gain : Gain  Gain=0.104667  OutDataTypeStr=Inherit: Same as input
  Gain1 : Gain  Gain=0.104667  OutDataTypeStr=Inherit: Same as input
  Gain4 : Gain  Gain=-1
  Gain6 : Gain  Gain=-1
  Logical Operator : Logic  Operator=OR  AllPortsSameDT=off  OutDataTypeStr=boolean
  Logical Operator1 : Logic  Inputs=3  AllPortsSameDT=off  OutDataTypeStr=boolean
  Logical Operator2 : Logic  Operator=OR  AllPortsSameDT=off  OutDataTypeStr=boolean
  Logical Operator3 : Logic  Inputs=3  AllPortsSameDT=off  OutDataTypeStr=boolean
  Logical Operator4 : Logic  Operator=OR  AllPortsSameDT=off  OutDataTypeStr=boolean
  Mux : Mux  Inputs=3
  Product{,1..3,6..9} (8 alike) : Product
  Product4 : Product  Inputs=4  OutDataTypeStr=single
  Product5 : Product  Inputs=3  OutDataTypeStr=single
  Relational Operator : RelationalOperator  Operator=~=  OutDataTypeStr=boolean  RndMeth=Simplest  InputSameDT=off
  Relational Operator1 : RelationalOperator  Operator=~=  OutDataTypeStr=boolean  RndMeth=Simplest  InputSameDT=off
  Relational Operator2 : RelationalOperator  Operator=~=  OutDataTypeStr=boolean  RndMeth=Simplest  InputSameDT=off
  Relational Operator3 : RelationalOperator  Operator=<  OutDataTypeStr=boolean  RndMeth=Simplest  InputSameDT=off
  Relational Operator4 : RelationalOperator  Operator=<  OutDataTypeStr=boolean  RndMeth=Simplest  InputSameDT=off
  Relational Operator5 : RelationalOperator  Operator=<  OutDataTypeStr=boolean  RndMeth=Simplest  InputSameDT=off
  Saturation Dynamic{,2..3,5} (4 alike) : simulink/Discontinuities/Saturation Dynamic  OutMin=[]  OutMax=[]  OutDataTypeStr=Inherit: Same as second input  OutDataType=fixdt(1, 16)  OutScaling=2^-10  DoSatur=off
  Unit Delay : UnitDelay  SampleTime=-1  HasFrameUpgradeWarning=on
  Unit Delay1 : UnitDelay  SampleTime=-1  HasFrameUpgradeWarning=on
  CCM_uQVoltTar : Outport  OutDataTypeStr=single  VectorParamsAs1DForOutWhenUnconnected=off
  CCM_uAlphaVoltTar : Outport  Port=2  OutDataTypeStr=single  VectorParamsAs1DForOutWhenUnconnected=off
  CCM_uBetaVoltTar : Outport  Port=3  OutDataTypeStr=single  VectorParamsAs1DForOutWhenUnconnected=off
  wires:
  Add3/1 -> CurrM_iDCurrSpdLopTarswt2/3
  Add5/1 -> Saturation Dynamic2/2  "CCM_uQVoltTarRaw"
  [CCM_bRstPI] -> CurrM_iDCurrSpdLopTarswt2/2
  [CurrM_iDCurrTar] -> Add/1
  Product2/1 -> Add5/1  "CCM_uQVoltTarKp"
  Constant13/1 -> CurrM_iDCurrSpdLopTarswt2/1
  Constant1/1 -> CurrM_iDCurrSpdLopTarswt3/1
  CCM_uQVoltTarswt/1 -> Saturation Dynamic5/2, Mux/3
  Constant12/1 -> CurrM_iDCurrSpdLopTarswt1/1
  Dead Zone Dynamic/1 -> Product/2, Product1/2  "CCM_iDCurrDiff"
  CurrM_iDCurrSpdLopTarswt3/1 -> Add4/2
  Dead Zone Dynamic1/1 -> Product2/2, Product3/2  "CCM_iQCurrDiff"
  [RotS_nRot] -> CCM_facCCMKpUqTar_T/1
  OpMod_stMotAct/1 -> Relational Operator2/1, Relational Operator1/1, Relational Operator/1  "OpMod_stMotAct"
  Constant3/1 -> Saturation Dynamic/3
  Relational Operator3/1 -> Logical Operator1/1
  Enumerated Constant/1 -> Relational Operator/2
  Abs3/1 -> Relational Operator5/1
  Constant15/1 -> Relational Operator5/2
  [CCM_bRstPI] -> CurrM_iDCurrSpdLopTarswt1/2
  CurrM_iDCurrTar/1 -> [CurrM_iDCurrTar], Abs1/1
  Constant9/1 -> Saturation Dynamic2/3
  CurrM_iQCurrTar/1 -> [CurrM_iQCurrTar], Abs2/1
  Add2/1 -> Saturation Dynamic/2  "CCM_uDVoltTarRaw"
  RotS_nRot/1 -> [RotS_nRot], Abs3/1  "RotS_nRot"
  Saturation Dynamic2/1 -> CCM_uQVoltTarswt/3
  CCM_facCCMKpUdTar_T/1 -> Product/1  "CCM_facCCMKpUd"
  Logical Operator2/1 -> [CCM_bRstPI]
  [CurrM_iQCurrTar] -> Add3/1
  Product1/1 -> Add1/1
  CurrM_iDCurrSpdLopTarswt4/1 -> Add1/2
  CCM_uDVoltTarTrig_C/1 -> CCM_uDVoltTarswt/2
  [RotS_nRot] -> CCM_facCCMKpUdTar_T/1
  Mux/1 -> Fcn/1, Fcn1/1
  Saturation Dynamic/1 -> CCM_uDVoltTarswt/3
  Unit Delay/1 -> CurrM_iDCurrSpdLopTarswt3/3
  Product7/1 -> Product5/1
  Fcn/1 -> CCM_uAlphaVoltTar/1
  Gain/1 -> Product8/1
  CurrM_iDCurrSpdLopTarswt7/1 -> Add2/3
  CurrM_iDCurrSpdLopTarswt6/1 -> Add5/3
  Constant22/1 -> CurrM_iDCurrSpdLopTarswt7/1
  CCM_uDVoltTarMor_C/1 -> CCM_uDVoltTarswt/1
  Relational Operator5/1 -> Logical Operator1/2
  CurrM_iDCurrSpdLopTarswt1/1 -> Dead Zone Dynamic/2  "CCM_iDCurrDiffRaw"
  Add1/1 -> Unit Delay1/1, Add2/2  "CCM_uDVoltTarKi"
  Constant21/1 -> CurrM_iDCurrSpdLopTarswt6/1
  [RotS_nRot] -> Gain/1
  CCM_uQVoltTarTrig_C/1 -> CCM_uQVoltTarswt/2
  Product8/1 -> Product4/1
  CCM_tqMotTarTrig_C5/1 -> Product8/2
  Product4/1 -> CurrM_iDCurrSpdLopTarswt7/3  "CCM_uDVoltTarVolFF"
  CCM_iQCurrAct/1 -> [CCM_iQCurrAct], Add3/2
  Constant17/1 -> Product4/4
  Abs1/1 -> Relational Operator3/1
  [CCM_iQCurrAct] -> Product4/3
  CCM_tqMotTarTrig_C2/1 -> Dead Zone Dynamic1/3
  [CCM_bRstPI] -> CurrM_iDCurrSpdLopTarswt7/2
  [CCM_iDCurrAct] -> Product6/2
  Constant8/1 -> Saturation Dynamic2/1
  CurrM_iDCurrSpdLopTarswt2/1 -> Dead Zone Dynamic1/2  "CCM_iQCurrDiffRaw"
  CCM_facCCMKiUdTar_T/1 -> Product1/1  "CCM_facCCMKiUd"
  CCM_uDVoltTarswt/1 -> Mux/2
  Relational Operator4/1 -> Logical Operator1/3
  CCM_tqMotTarTrig_C3/1 -> Product7/2
  Product5/1 -> CurrM_iDCurrSpdLopTarswt6/3  "CCM_uQVoltTarVolFF"
  CCM_facCCMKiUqTar_T/1 -> Product3/1  "CCM_facCCMKiUq"
  Unit Delay1/1 -> CurrM_iDCurrSpdLopTarswt4/3
  CCM_tqMotTarTrig_C1/1 -> Dead Zone Dynamic1/1
  Constant19/1 -> Product5/2
  Fcn1/1 -> CCM_uBetaVoltTar/1
  Abs2/1 -> Relational Operator4/1
  Product6/1 -> Add6/1
  CCM_facCCMKpUqTar_T/1 -> Product2/1  "CCM_facCCMKpUq"
  Add6/1 -> Product5/3
  CCM_uQVoltTarMor_C/1 -> CCM_uQVoltTarswt/1
  CCM_tqMotTarTrig_C8/1 -> Dead Zone Dynamic/3
  Gain1/1 -> Product7/1
  Constant2/1 -> Saturation Dynamic/1
  CCM_iDCurrAct/1 -> [CCM_iDCurrAct], Add/2
  RotS_agRot/1 -> Add7/2
  [RotS_nRot] -> Gain1/1
  CCM_tqMotTarTrig_C7/1 -> Dead Zone Dynamic/1
  [CCM_bRstPI] -> CurrM_iDCurrSpdLopTarswt6/2
  Add/1 -> CurrM_iDCurrSpdLopTarswt1/3
  Logical Operator1/1 -> CCM_uDVoltTarswt1/3
  Product3/1 -> Add4/1
  CCM_tqMotTarTrig_C4/1 -> Add6/2
  [RotS_nRot] -> CCM_facCCMKiUdTar_T/1
  [RotS_nRot] -> CCM_facCCMKiUqTar_T/1
  Product/1 -> Add2/1  "CCM_uDVoltTarKp"
  Constant14/1 -> Relational Operator4/2
  Constant4/1 -> CurrM_iDCurrSpdLopTarswt4/1
  Constant5/1 -> Relational Operator3/2
  Enumerated Constant1/1 -> Relational Operator1/2
  Enumerated Constant2/1 -> Relational Operator2/2
  Relational Operator1/1 -> Logical Operator3/2
  Relational Operator/1 -> Logical Operator3/1
  Relational Operator2/1 -> Logical Operator3/3
  Logical Operator3/1 -> Logical Operator2/1
  [CCM_bRstPI] -> Logical Operator/1
  Logical Operator/1 -> CurrM_iDCurrSpdLopTarswt4/2
  CCM_tqMotTarTrig_C6/1 -> Logical Operator/2
  CCM_tqMotTarTrig_C9/1 -> Logical Operator4/2
  Logical Operator4/1 -> CurrM_iDCurrSpdLopTarswt3/2
  [CCM_bRstPI] -> Logical Operator4/1
  CCM_uDVoltTarTrig_C1/1 -> CCM_uDVoltTarswt1/2
  CCM_uDVoltTarMor_C1/1 -> CCM_uDVoltTarswt1/1
  CCM_uDVoltTarswt1/1 -> Logical Operator2/2
  Constant6/1 -> Product9/1
  Product9/1 -> Add7/1
  Add7/1 -> Mux/1
  Saturation Dynamic5/1 -> CCM_uQVoltTar/1  "CCM_uQVoltTar"
  Saturation Dynamic3/1 -> Unit Delay/1, Add5/2  "CCM_uDVoltTarKi"
  ? -> Saturation Dynamic5/1
  ? -> Gain4/1
  Gain4/1 -> Saturation Dynamic5/3
  [DSS_uPhaseLim] -> Saturation Dynamic3/1
  Gain6/1 -> Saturation Dynamic3/3
  [DSS_uPhaseLim] -> Gain6/1
  Add4/1 -> Saturation Dynamic3/2  "CCM_uDVoltTarKiaw"
  RotS_radRot/1 -> Product9/2
  [CCM_iQCurrAct] -> CCM_facCCMLq_T/2
  [CCM_iDCurrAct] -> CCM_facCCMLq_T/1
  CCM_facCCMLq_T/1 -> Product4/2
  [CCM_iDCurrAct] -> CCM_facCCMLd_T/1
  [CCM_iQCurrAct] -> CCM_facCCMLd_T/2
  CCM_facCCMLd_T/1 -> Product6/1

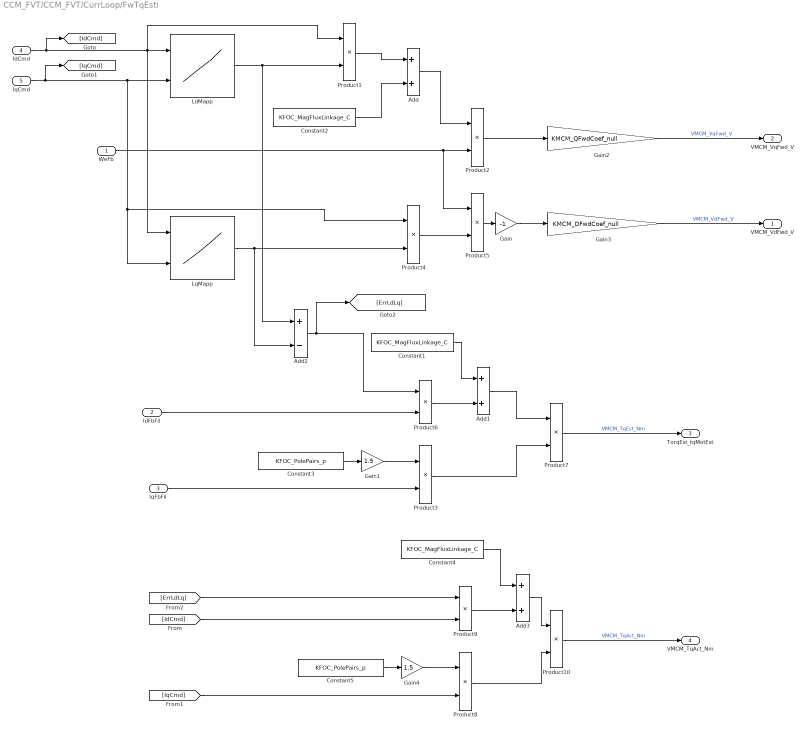
== system CCM_FVT/CCM_FVT/CurrLoop/FwTqEsti ==
  WeFb : Inport
  IdFbFil : Inport  Port=2
  IqFbFil : Inport  Port=3
  IdCmd : Inport  Port=4
  IqCmd : Inport  Port=5
  Add : Sum
  Add1 : Sum
  Add2 : Sum  Inputs=+-
  Add3 : Sum
  Constant1 : Constant  Value=KFOC_MagFluxLinkage_C  OutDataTypeStr=single
  Constant2 : Constant  Value=KFOC_MagFluxLinkage_C  OutDataTypeStr=single
  Constant3 : Constant  Value=KFOC_PolePairs_p  OutDataTypeStr=single
  Constant4 : Constant  Value=KFOC_MagFluxLinkage_C  OutDataTypeStr=single
  Constant5 : Constant  Value=KFOC_PolePairs_p  OutDataTypeStr=single
  Gain : Gain  Gain=-1
  Gain1 : Gain  Gain=1.5
  Gain2 : Gain  Gain=KMCM_QFwdCoef_null
  Gain3 : Gain  Gain=KMCM_DFwdCoef_null
  Gain4 : Gain  Gain=1.5
  LdMapp : Lookup_n-D  BreakpointsForDimension1=ACCM_facCCMLq_Y_A  BreakpointsForDimension2=ACCM_facCCMLq_X_A  Table=MCCM_facCCMLd_Z_T  ExtrapMethod=Clip  UseLastTableValue=on  InternalRulePriority=Speed  RndMeth=Simplest
      settings: InputPortMap=u0,u1
  LqMapp : Lookup_n-D  BreakpointsForDimension1=ACCM_facCCMLq_Y_A  BreakpointsForDimension2=ACCM_facCCMLq_X_A  Table=MCCM_facCCMLq_Z_T  ExtrapMethod=Clip  UseLastTableValue=on  InternalRulePriority=Speed  RndMeth=Simplest
      settings: InputPortMap=u0,u1
  Product{1..10} (10 alike) : Product  RndMeth=Zero
  VMCM_VdFwd_V : Outport
  VMCM_VqFwd_V : Outport  Port=2
  TorqEst_tqMotEst : Outport  Port=3
  VMCM_TqAct_Nm : Outport  Port=4
  wires:
  Product2/1 -> Gain2/1
  Gain/1 -> Gain3/1
  Product4/1 -> Product5/2
  Product5/1 -> Gain/1
  Product1/1 -> Add/1
  Add/1 -> Product2/1
  Constant3/1 -> Gain1/1
  Gain1/1 -> Product3/1
  Product6/1 -> Add1/2
  Add1/1 -> Product7/1
  Product3/1 -> Product7/2
  Product7/1 -> TorqEst_tqMotEst/1  "VMCM_TqEst_Nm"
  Gain2/1 -> VMCM_VqFwd_V/1  "VMCM_VqFwd_V"
  Gain3/1 -> VMCM_VdFwd_V/1  "VMCM_VdFwd_V"
  IdCmd/1 -> [IdCmd], LqMapp/1, LdMapp/1, Product1/1
  IqCmd/1 -> [IqCmd], LdMapp/2, LqMapp/2, Product4/1
  Constant2/1 -> Add/2
  LdMapp/1 -> Add2/1, Product1/2
  WeFb/1 -> Product5/1, Product2/2
  LqMapp/1 -> Add2/2, Product4/2
  IdFbFil/1 -> Product6/2
  Add2/1 -> [ErrLdLq], Product6/1
  Constant1/1 -> Add1/1
  IqFbFil/1 -> Product3/2
  [IqCmd] -> Product8/2
  Constant4/1 -> Add3/1
  [ErrLdLq] -> Product9/1
  [IdCmd] -> Product9/2
  Product10/1 -> VMCM_TqAct_Nm/1  "VMCM_TqAct_Nm"
  Product8/1 -> Product10/2
  Add3/1 -> Product10/1
  Product9/1 -> Add3/2
  Gain4/1 -> Product8/1
  Constant5/1 -> Gain4/1

== system CCM_FVT/CCM_FVT/CurrLoop/Harmonic Inject ==
  "VCCM_VdTmp_V " : Inport
  VCCM_VqTmp_V : Inport  Port=2
  "Omega " : Inport  Port=3
  "Torque " : Inport  Port=4
  12Orfer Harmonic Inject : Subsystem
  6Order Harmonic Inject : Subsystem
  Sum : Sum  Inputs=|++
  Sum1 : Sum  Inputs=|++
  "VHJM_VdCmd_V " : Outport  VectorParamsAs1DForOutWhenUnconnected=off
  "VHJM_VqCmd_V " : Outport  Port=2  VectorParamsAs1DForOutWhenUnconnected=off
  wires:
  "Torque "/1 -> 12Orfer Harmonic Inject/1("Torque "), 6Order Harmonic Inject/1("Torque ")
  6Order Harmonic Inject/1("Vd ") -> Sum/1
  "VCCM_VdTmp_V "/1 -> Sum/2
  12Orfer Harmonic Inject/1("Vq ") -> Sum1/1
  VCCM_VqTmp_V/1 -> Sum1/2
  Sum/1 -> "VHJM_VdCmd_V "/1
  Sum1/1 -> "VHJM_VqCmd_V "/1
  "Omega "/1 -> 12Orfer Harmonic Inject/2("Omega "), 6Order Harmonic Inject/2("Omega ")

== system CCM_FVT/CCM_FVT/CurrLoop/PI ==
  VCCM_IqCmd_A : Inport
  VCCM_IdCmd_A : Inport  Port=2
  VCCM_VdCmd _V : Inport  Port=3
  VCCM_IdFb_A : Inport  Port=4
  VCCM_VdFwd_V : Inport  Port=5
  VCCM_IqFb_A : Inport  Port=6
  VCCM_VqFwd_V : Inport  Port=7
  VCCM_VqCmd_V : Inport  Port=8
  RotS_nRot : Inport  Port=9  OutDataTypeStr=single
  CurLoopEna : Inport  Port=10
  IdPI : Subsystem
  IqPI : Subsystem
  VCCM_VdRef_V : Outport  VectorParamsAs1DForOutWhenUnconnected=off
  VCCM_VqRef_V : Outport  Port=2  VectorParamsAs1DForOutWhenUnconnected=off
  wires:
  CurLoopEna/1 -> IqPI/2(CurLoopActEna), IdPI/5(CurLoopActEna)
  VCCM_VqFwd_V/1 -> IqPI/5(VqFwd)
  VCCM_IqFb_A/1 -> IqPI/4(IqFb)
  VCCM_IdFb_A/1 -> IdPI/3(IdFb)
  VCCM_VdFwd_V/1 -> IdPI/4(VdFwd)
  VCCM_VqCmd_V/1 -> IqPI/6(VqLim)
  IqPI/1(VqRef) -> VCCM_VqRef_V/1  "VCCM_VqRef_V"
  VCCM_IdCmd_A/1 -> IdPI/2(IdCmd)
  VCCM_IqCmd_A/1 -> IqPI/3(IqCmd)
  VCCM_VdCmd _V/1 -> IdPI/1(VdLim)
  IdPI/1(VdRef) -> VCCM_VdRef_V/1  "VCCM_VdRef_V"
  RotS_nRot/1 -> IqPI/1("SpdFil "), IdPI/6("SpdFil ")

== system CCM_FVT/CCM_FVT/CurrLoop/RCM ==
  "Reset " : Inport
  "VCCM_VdCmd_V " : Inport  Port=2
  "VCCM_IdFb_A " : Inport  Port=3
  "VCCM_VqCmd_V " : Inport  Port=4
  "VCCM_IqFb_A " : Inport  Port=5
  Enable : EnablePort  StatesWhenEnabling=reset
  Constant : Constant  Value=KRCM_SeleDAxes_flg
  Subsystem : Subsystem
  Switch1 : Switch  Criteria=u2 ~= 0  SaturateOnIntegerOverflow=off  InputSameDT=off
  Switch2 : Switch  Criteria=u2 ~= 0  SaturateOnIntegerOverflow=off  InputSameDT=off
  "VRCM_RsvLrnAngle_rad " : Outport  VectorParamsAs1DForOutWhenUnconnected=off
  wires:
  Subsystem/1("VRCM_RsvLrnAngle_rad ") -> "VRCM_RsvLrnAngle_rad "/1
  Switch1/1 -> Subsystem/1("VCCM_VoltCmd_V ")
  Switch2/1 -> Subsystem/2("VCCM_CurFb_A ")
  "VCCM_VdCmd_V "/1 -> Switch1/1
  "VCCM_IdFb_A "/1 -> Switch2/1
  "VCCM_VqCmd_V "/1 -> Switch1/3
  "VCCM_IqFb_A "/1 -> Switch2/3
  Constant/1 -> Switch1/2, Switch2/2
  "Reset "/1 -> Subsystem/3("Reset ")

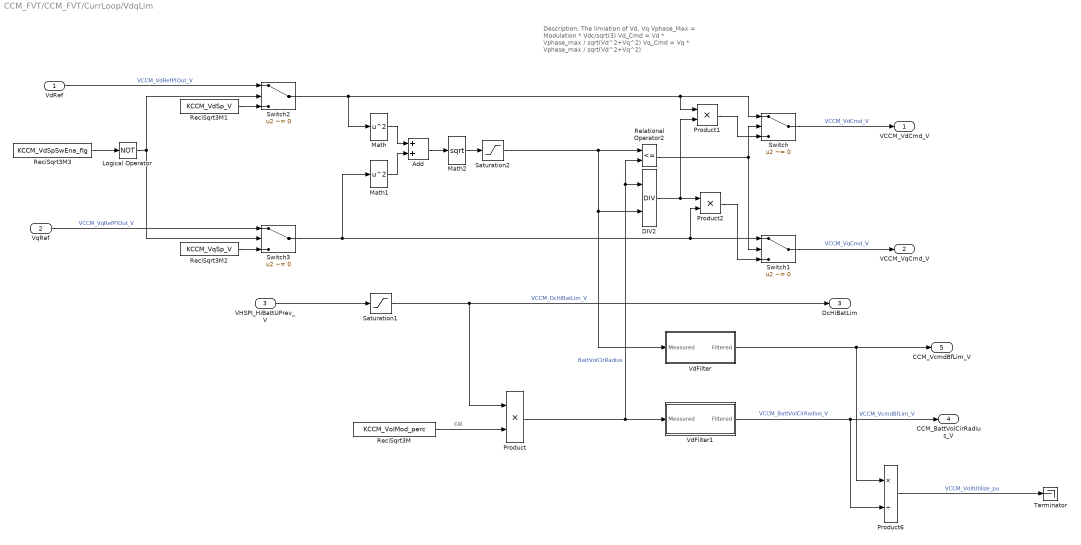
== system CCM_FVT/CCM_FVT/CurrLoop/VdqLim ==
  note: Description:
      | The limiation of Vd, Vq
      | Vphase_Max = Modulation * Vdc/sqrt(3)
      | Vd_Cmd = Vd * Vphase_max / sqrt(Vd^2+Vq^2)
      | Vq_Cmd = Vq * Vphase_max / sqrt(Vd^2+Vq^2)
  note: cal
  VdRef : Inport
  VqRef : Inport  Port=2
  VHSPI_HiBattUPrev_V : Inport  Port=3
  Add : Sum
  DIV2 : GRC_Lib/ArithmeticOperations/DIV  MinDivVal=1e-15  IpDT=single
  Logical Operator : Logic  Operator=NOT  AllPortsSameDT=off  OutDataTypeStr=boolean
  Math : Math  Operator=square  SignedPower=on
  Math1 : Math  Operator=square  SignedPower=on
  Math2 : Math  Operator=sqrt  SignedPower=on
  Product : Product  Inputs=**  RndMeth=Zero
  Product1 : Product  RndMeth=Zero
  Product2 : Product  RndMeth=Zero
  Product6 : Product  Inputs=*/  RndMeth=Zero  OutDataTypeStr=Inherit: Same as first input
  ReciSqrt3M : Constant  Value=KCCM_VolMod_perc  OutDataTypeStr=single
  ReciSqrt3M1 : Constant  Value=KCCM_VdSp_V  OutDataTypeStr=single
  ReciSqrt3M2 : Constant  Value=KCCM_VqSp_V  OutDataTypeStr=single
  ReciSqrt3M3 : Constant  Value=KCCM_VdSpSwEna_flg  OutDataTypeStr=single
  Relational Operator2 : RelationalOperator  Operator=<=  OutDataTypeStr=boolean  InputSameDT=off
  Saturation1 : Saturate  UpperLimit=1023  LowerLimit=1
      settings: AttributesFormatString=|
      | UpperLimit : %<UpperLimit>
      | LowerLimit : %<LowerLimit>
  Saturation2 : Saturate  UpperLimit=1023  LowerLimit=1
      settings: AttributesFormatString=|
      | UpperLimit : %<UpperLimit>
      | LowerLimit : %<LowerLimit>
  Switch{,1..3} (4 alike) : Switch  Criteria=u2 ~= 0  SaturateOnIntegerOverflow=off  InputSameDT=off
      settings: AttributesFormatString=%<Criteria>
  Terminator : Terminator
  VdFilter : Subsystem
  VdFilter1 : Subsystem
  VCCM_VdCmd_V : Outport
  VCCM_VqCmd_V : Outport  Port=2
  DcHiBatLim : Outport  Port=3
  CCM_BattVolCirRadius_V : Outport  Port=4
  CCM_VcmdBfLim_V : Outport  Port=5
  wires:
  VdFilter/1(Filtered) -> Product6/1, CCM_VcmdBfLim_V/1  "VCCM_VcmdBfLim_V"
  VdFilter1/1(Filtered) -> Product6/2, CCM_BattVolCirRadius_V/1  "VCCM_BattVolCirRadius_V"
  Product2/1 -> Switch1/3
  Product1/1 -> Switch/3
  Product/1 -> VdFilter1/1(Measured), DIV2/1, Relational Operator2/2  "BattVolCirRadius"
  ReciSqrt3M/1 -> Product/2
  Saturation1/1 -> Product/1, DcHiBatLim/1  "VCCM_DcHiBatLim_V"
  DIV2/1 -> Product2/1, Product1/2
  Relational Operator2/1 -> Switch1/2, Switch/2
  Add/1 -> Math2/1
  Switch/1 -> VCCM_VdCmd_V/1  "VCCM_VdCmd_V"
  Switch1/1 -> VCCM_VqCmd_V/1  "VCCM_VqCmd_V"
  Math1/1 -> Add/2
  Math/1 -> Add/1
  Math2/1 -> Saturation2/1
  VHSPI_HiBattUPrev_V/1 -> Saturation1/1
  Saturation2/1 -> DIV2/2, VdFilter/1(Measured), Relational Operator2/1
  ReciSqrt3M3/1 -> Logical Operator/1
  Switch2/1 -> Product1/1, Switch/1, Math/1
  Switch3/1 -> Product2/2, Switch1/1, Math1/1
  VqRef/1 -> Switch3/1  "VCCM_VqRefPIOut_V"
  ReciSqrt3M2/1 -> Switch3/3
  ReciSqrt3M1/1 -> Switch2/3
  Logical Operator/1 -> Switch2/2, Switch3/2
  Product6/1 -> Terminator/1  "VCCM_VoltUtilize_pu"
  VdRef/1 -> Switch2/1  "VCCM_VdRefPIOut_V"

== system CCM_FVT/CCM_FVT/CurrLoop/ASCCal/If Action Subsystem ==
  VdRef : Inport
  VqRef : Inport  Port=2
  ASCFlag : Inport  Port=3
  Action Port : ActionPort
  Vd : Outport
  Vq : Outport  Port=2
  enASC_flg : Outport  Port=3
  wires:
  VdRef/1 -> Vd/1
  VqRef/1 -> Vq/1
  ASCFlag/1 -> enASC_flg/1

== system CCM_FVT/CCM_FVT/CurrLoop/ASCCal/Subsystem1 ==
  VdRef : Inport
  VqRef : Inport  Port=2
  "ASCFlag " : Inport  Port=3
  Action Port : ActionPort
  Constant1 : Constant  Value=KCCM_UdqASCTimesValue_C  OutDataTypeStr=single  SampleTime=-1
  Constant3 : Constant  Value=KCCM_UdqASCTagValue_C  OutDataTypeStr=single  SampleTime=-1
  Ramp : Stateflow chart  TreatAsAtomicUnit=on
  Vd : Outport
  Vq : Outport  Port=2
  enASC_flg : Outport  Port=3
  wires:
  Ramp/2(intVq) -> Vq/1
  Ramp/1(intVd) -> Vd/1
  VqRef/1 -> Ramp/2(Vq)
  VdRef/1 -> Ramp/1(Vd)
  "ASCFlag "/1 -> Ramp/3(enableTrajGen_flg)
  Ramp/3(enASC_flg) -> enASC_flg/1
  Constant1/1 -> Ramp/5(times)
  Constant3/1 -> Ramp/4(targetValue)

== system CCM_FVT/CCM_FVT/CurrLoop/ActCurrDQ/UvToDq ==
  PosnCur : Inport
  PhaUCur : Inport  Port=2
  PhaVCur : Inport  Port=3
  Action Port : ActionPort
  Clarke_Function : Subsystem
  Constant1 : Constant  Commented=on  Value=KCCM_PosnRange_deg  OutDataTypeStr=single
  Park_Function : Subsystem
  Sin : Trigonometry
  Sin1 : Trigonometry  Operator=cos
  TriAgTbl : Subsystem  Commented=on
      settings: RTWFcnNameOpts=Use subsystem name
  IdFb : Outport
  IqFb : Outport  Port=2
  wires:
  Park_Function/1(IqFb) -> IqFb/1
  Park_Function/2(IdFb) -> IdFb/1
  Clarke_Function/1(IalphaFb) -> Park_Function/1(IalphaFb)
  Clarke_Function/2(IbetaFb) -> Park_Function/2(IbetaFb)
  Sin1/1 -> Park_Function/4(Cos)
  PhaUCur/1 -> Clarke_Function/1(PhaUCur)
  PhaVCur/1 -> Clarke_Function/2(PhaVCur)
  PosnCur/1 -> Sin1/1, Sin/1
  Sin/1 -> Park_Function/3(Sin)
  Constant1/1 -> TriAgTbl/2(PosnRange)

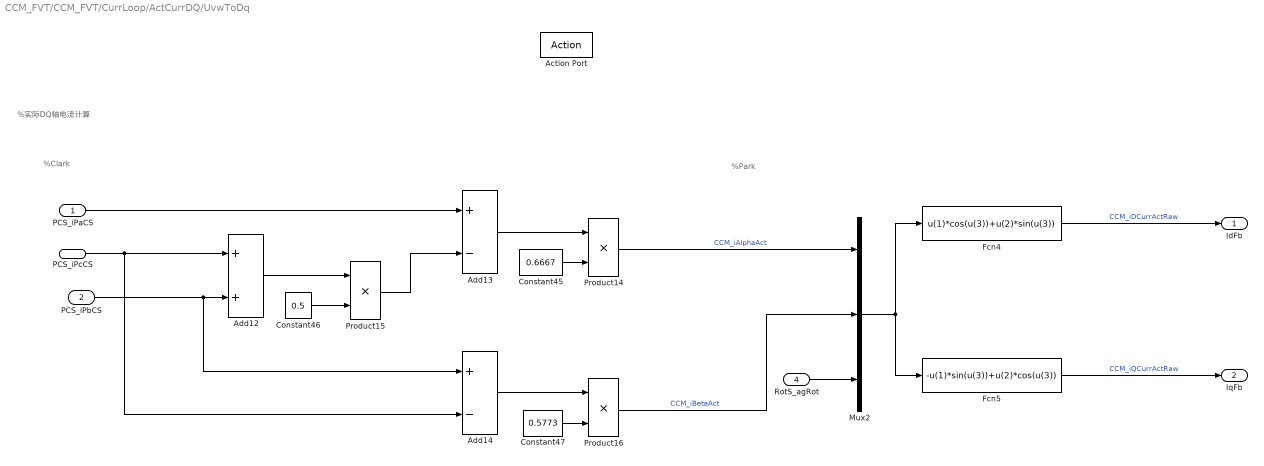
== system CCM_FVT/CCM_FVT/CurrLoop/ActCurrDQ/UvwToDq ==
  note: %实际DQ轴电流计算
  note: %Park
  note: %Clark
  PCS_iPaCS : Inport  OutDataTypeStr=single
  PCS_iPbCS : Inport  Port=2  OutDataTypeStr=single
  PCS_iPcCS : Inport  Port=3  OutDataTypeStr=single
  RotS_agRot : Inport  Port=4  OutDataTypeStr=single
  Action Port : ActionPort
  Add12 : Sum
  Add13 : Sum  Inputs=+-
  Add14 : Sum  Inputs=+-
  Constant45 : Constant  Value=0.6667  OutDataTypeStr=single
  Constant46 : Constant  Value=0.5  OutDataTypeStr=single
  Constant47 : Constant  Value=0.5773  OutDataTypeStr=single
  Fcn4 : Fcn  Expr=u(1)*cos(u(3))+u(2)*sin(u(3))
  Fcn5 : Fcn  Expr=-u(1)*sin(u(3))+u(2)*cos(u(3))
  Mux2 : Mux  Inputs=3
  Product14 : Product
  Product15 : Product
  Product16 : Product
  IdFb : Outport
  IqFb : Outport  Port=2
  wires:
  Fcn5/1 -> IqFb/1  "CCM_iQCurrActRaw"
  Mux2/1 -> Fcn5/1, Fcn4/1
  Constant46/1 -> Product15/2
  PCS_iPcCS/1 -> Add14/2, Add12/1
  Product14/1 -> Mux2/1  "CCM_iAlphaAct"
  PCS_iPbCS/1 -> Add14/1, Add12/2
  Add14/1 -> Product16/1
  Product16/1 -> Mux2/2  "CCM_iBetaAct"
  Product15/1 -> Add13/2
  Add13/1 -> Product14/1
  Constant47/1 -> Product16/2
  Add12/1 -> Product15/1
  Fcn4/1 -> IdFb/1  "CCM_iDCurrActRaw"
  PCS_iPaCS/1 -> Add13/1
  RotS_agRot/1 -> Mux2/3
  Constant45/1 -> Product14/2

== system CCM_FVT/CCM_FVT/CurrLoop/Harmonic Inject/12Orfer Harmonic Inject ==
  "Torque " : Inport
  "Omega " : Inport  Port=2
  Add : Sum  OutDataTypeStr=Inherit: Same as first input
  "Amplitude " : Lookup_n-D  NumberOfTableDimensions=1  BreakpointsForDimension1=MHJM_TrqRefX_Nm  Table=MHJM_Order12AmpY_A  ExtrapMethod=Clip  UseLastTableValue=on  InternalRulePriority=Speed  RndMeth=Simplest
  Gain : Gain  Gain=KHJM_EnaOrd12HJ_value
  Gain1 : Gain  Gain=12  OutDataTypeStr=Inherit: Same as input
  Ki2 : Constant  Value=KCCM_CurLoopPrd_t  SampleTime=-1
  "Phase " : Lookup_n-D  NumberOfTableDimensions=1  BreakpointsForDimension1=MHJM_TrqRefX_Nm  Table=MHJM_Order12PhaseY_rad  ExtrapMethod=Clip  UseLastTableValue=on  InternalRulePriority=Speed  RndMeth=Simplest
  Product : Product
  Product1 : Product
  Sin : Trigonometry
  "Vq " : Outport  VectorParamsAs1DForOutWhenUnconnected=off
  wires:
  Ki2/1 -> Product1/2
  "Torque "/1 -> "Phase "/1, "Amplitude "/1
  Sin/1 -> Product/2
  Product/1 -> Gain/1
  "Omega "/1 -> Product1/1
  Add/1 -> Sin/1
  Gain/1 -> "Vq "/1  "VHJM_Order12Vd_V"
  Product1/1 -> Gain1/1
  "Amplitude "/1 -> Product/1
  "Phase "/1 -> Add/1
  Gain1/1 -> Add/2

== system CCM_FVT/CCM_FVT/CurrLoop/Harmonic Inject/6Order Harmonic Inject ==
  "Torque " : Inport
  "Omega " : Inport  Port=2
  Add : Sum  OutDataTypeStr=Inherit: Same as first input
  "Amplitude " : Lookup_n-D  NumberOfTableDimensions=1  BreakpointsForDimension1=MHJM_TrqRefX_Nm  Table=MHJM_Order6AmpY_A  ExtrapMethod=Clip  UseLastTableValue=on  InternalRulePriority=Speed  RndMeth=Simplest
  Gain : Gain  Gain=KHJM_EnaOrd6HJ_value
  Gain1 : Gain  Gain=6  OutDataTypeStr=Inherit: Same as input
  Ki2 : Constant  Value=KCCM_CurLoopPrd_t  SampleTime=-1
  "Phase " : Lookup_n-D  NumberOfTableDimensions=1  BreakpointsForDimension1=MHJM_TrqRefX_Nm  Table=MHJM_Order6PhaseY_rad  ExtrapMethod=Clip  UseLastTableValue=on  InternalRulePriority=Speed  RndMeth=Simplest
  Product : Product
  Product1 : Product
  Sin : Trigonometry
  "Vd " : Outport  VectorParamsAs1DForOutWhenUnconnected=off
  wires:
  "Phase "/1 -> Add/1
  "Amplitude "/1 -> Product/1
  Product1/1 -> Gain1/1
  Gain/1 -> "Vd "/1  "VHJM_Order6Vd_V"
  Add/1 -> Sin/1
  "Omega "/1 -> Product1/1
  Product/1 -> Gain/1
  Sin/1 -> Product/2
  "Torque "/1 -> "Amplitude "/1, "Phase "/1
  Ki2/1 -> Product1/2
  Gain1/1 -> Add/2

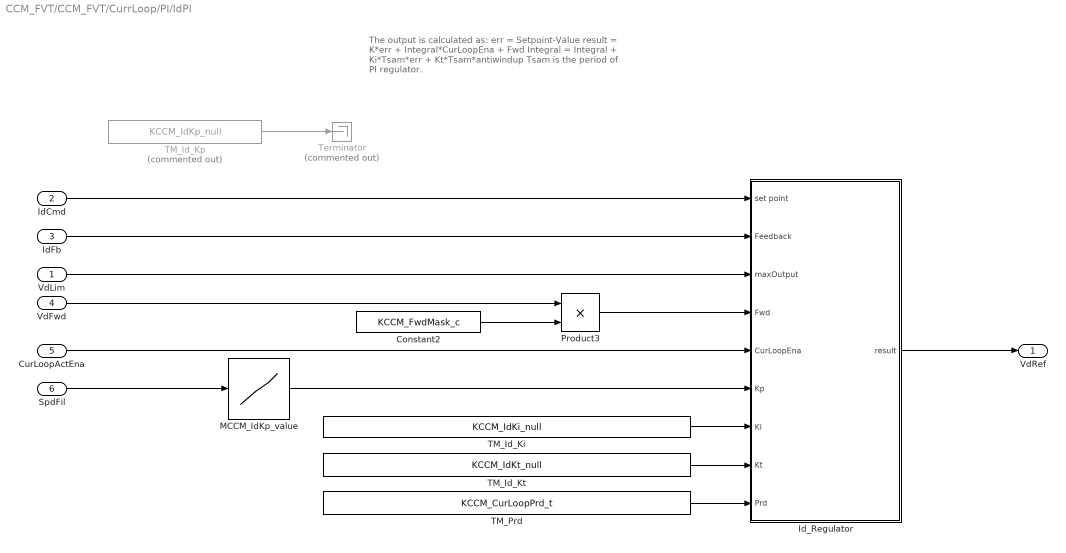
== system CCM_FVT/CCM_FVT/CurrLoop/PI/IdPI ==
  note: The output is calculated as:
      | err = Setpoint-Value
      | result = K*err + Integral*CurLoopEna + Fwd
      | Integral = Integral + Ki*Tsam*err + Kt*Tsam*antiwindup
      | Tsam is the period of PI regulator.
  VdLim : Inport
  IdCmd : Inport  Port=2
  IdFb : Inport  Port=3
  VdFwd : Inport  Port=4
  CurLoopActEna : Inport  Port=5
  "SpdFil " : Inport  Port=6
  Constant2 : Constant  Value=KCCM_FwdMask_c  OutDataTypeStr=single
  Id_Regulator : Subsystem
  MCCM_IdKp_value : Lookup_n-D  NumberOfTableDimensions=1  BreakpointsForDimension1=ACCM_IdKp_X_rpm  Table=MCCM_IdKp_Y_value  ExtrapMethod=Clip  UseLastTableValue=on  InternalRulePriority=Speed  RndMeth=Simplest
  Product3 : Product  Inputs=**  RndMeth=Zero
  TM_Id_Ki : Constant  Value=KCCM_IdKi_null  OutDataTypeStr=single
  TM_Id_Kp : Constant  Commented=on  Value=KCCM_IdKp_null  OutDataTypeStr=single
  TM_Id_Kt : Constant  Value=KCCM_IdKt_null  OutDataTypeStr=single
  TM_Prd : Constant  Value=KCCM_CurLoopPrd_t  OutDataTypeStr=single
  Terminator : Terminator  Commented=on
  VdRef : Outport
  wires:
  VdFwd/1 -> Product3/1
  Product3/1 -> Id_Regulator/4(Fwd)
  Constant2/1 -> Product3/2
  TM_Prd/1 -> Id_Regulator/9(Prd)
  TM_Id_Kt/1 -> Id_Regulator/8(Kt)
  TM_Id_Ki/1 -> Id_Regulator/7(Ki)
  VdLim/1 -> Id_Regulator/3(maxOutput)
  CurLoopActEna/1 -> Id_Regulator/5(CurLoopEna)
  IdFb/1 -> Id_Regulator/2(Feedback)
  IdCmd/1 -> Id_Regulator/1(set point)
  Id_Regulator/1(result) -> VdRef/1
  TM_Id_Kp/1 -> Terminator/1
  "SpdFil "/1 -> MCCM_IdKp_value/1
  MCCM_IdKp_value/1 -> Id_Regulator/6(Kp)
